simulink model "thrust_curve_test"  (R2014a)
settings: Solver=ode45  StartTime=0.0  StopTime=10.0  RelTol=1e-3
libraries: rocket_thrust_data_library x1
settings Model: Creator=scorpii  LastModifiedBy=scorpii

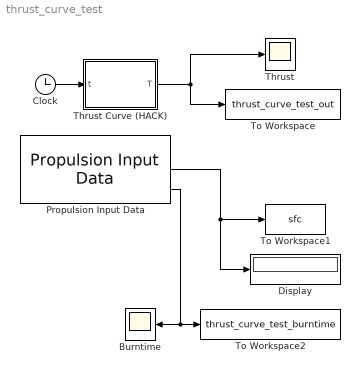
== system thrust_curve_test ==
  Burntime : Scope
  Clock : Clock
  Display : Display
  Propulsion Input Data : rocket_thrust_data_library/Propulsion Input Data
      link override Provided Specific Fuel Consumption: Value=0.0005387
  Thrust : Scope
  Thrust Curve (HACK) : MATLAB Function  TreatAsAtomicUnit=on
  To Workspace : ToWorkspace  VariableName=thrust_curve_test_out  SampleTime=-1
  To Workspace1 : ToWorkspace  VariableName=sfc  SampleTime=-1
  To Workspace2 : ToWorkspace  VariableName=thrust_curve_test_burntime  SampleTime=-1
  wires:
  Propulsion Input Data/2 -> Display/1, To Workspace1/1
  Propulsion Input Data/3 -> Burntime/1, To Workspace2/1
  Clock/1 -> Thrust Curve (HACK)/1(t)
  Thrust Curve (HACK)/1(T) -> Thrust/1, To Workspace/1

== matlab function thrust_curve_test/Thrust Curve (HACK) ==
  data: t input; T output
function T = thrust_hack(t)
    if t<0.08
    T=4000000*t^3-462933*t^2+41915*t+209.66
    elseif t<0.15935
    T=-4701*t+2748.7
    elseif t<0.21276 
    T=-1133.2*t+2223.6 
    elseif t<0.32775
    T=787.15*t+1850.2
    elseif t<0.57775
    T=-754.4*t+2339.9
    elseif t<0.72775
    T=-251*t+2070.7 
    elseif t<1.7277
    T=-70.147*t+1947.4
    elseif t<3.3777
    T=-31.421*t^2-9.1503*t+1930.8
    elseif t<3.9777
    T=3656.6*t^3-39167*t^2+137806*t-158018
    elseif t<4.5277
    T=-1051.8*t+4709.4
    else
    T=0
end
